simulink model "P1_ADR"  (R2020b)
settings: Solver=VariableStepAuto  StartTime=0.0  StopTime=40  RelTol=1e-3
undefined symbols (not defined in the file): DiscIntNeverNeededParam
libraries: simulink x1
settings Model: Creator=marta  LastModifiedBy=Danie

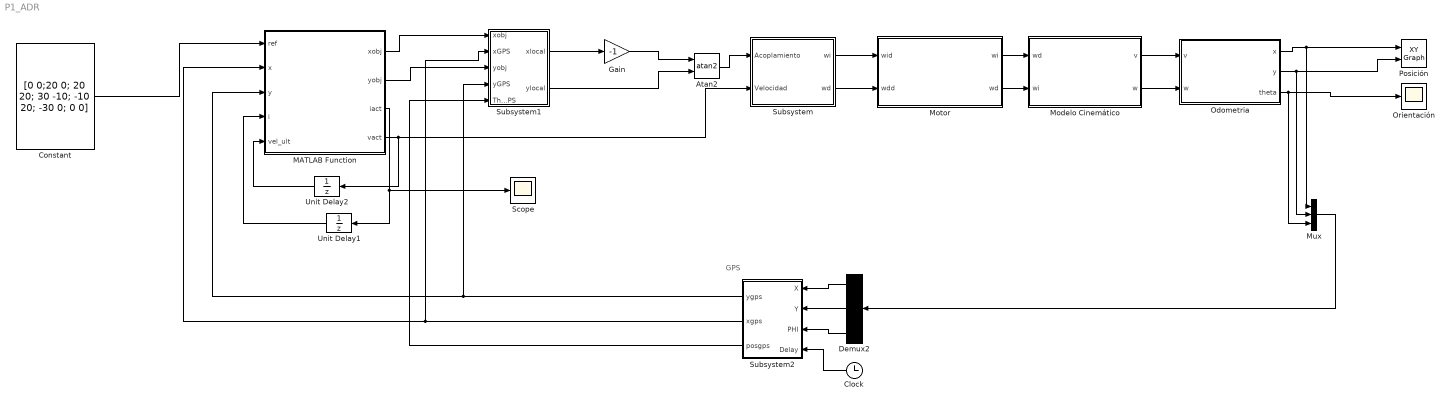
== system P1_ADR ==
  note: GPS
  Atan2 : Trigonometry  Operator=atan2
  Clock : Clock
  Constant : Constant  Value=[0 0;20 0; 20 20; 30 -10; -10 20; -30 0; 0 0]
  Demux2 : Demux  Outputs=3
  Gain : Gain  Gain=-1
  MATLAB Function : MATLAB Function  TreatAsAtomicUnit=on
  Modelo Cinemático : Subsystem
  Motor : Subsystem
  Mux : Mux  Inputs=3
  Odometria : Subsystem
  Orientación : Scope
  Posición : simulink/Sinks/XY Graph  xmin=-5  xmax=5  ymin=-40  ymax=40  st=-1
  Scope : Scope
  Subsystem : Subsystem
  Subsystem1 : Subsystem
  Subsystem2 : Subsystem
  Unit Delay1 : UnitDelay  SampleTime=-1  HasFrameUpgradeWarning=on
  Unit Delay2 : UnitDelay  SampleTime=-1  HasFrameUpgradeWarning=on
  wires:
  Modelo Cinemático/1(v) -> Odometria/1(v)
  Motor/1(wi) -> Modelo Cinemático/1(wd)
  Motor/2(wd) -> Modelo Cinemático/2(wi)
  Modelo Cinemático/2(w) -> Odometria/2(w)
  Odometria/1(x) -> Mux/1, Posición/1
  Odometria/2(y) -> Mux/2, Posición/2
  Odometria/3(theta) -> Mux/3, Orientación/1
  Constant/1 -> MATLAB Function/1(ref)
  MATLAB Function/3(iact) -> Unit Delay1/1, Scope/1
  Unit Delay1/1 -> MATLAB Function/4(i)
  MATLAB Function/1(xobj) -> Subsystem1/1(xobj)
  MATLAB Function/2(yobj) -> Subsystem1/3(yobj)
  Subsystem1/2(ylocal) -> Atan2/2
  Gain/1 -> Atan2/1
  Subsystem1/1(xlocal) -> Gain/1
  Atan2/1 -> Subsystem/1(Acoplamiento)
  Subsystem/2(wd) -> Motor/2(wdd)
  Subsystem/1(wi) -> Motor/1(wid)
  Mux/1 -> Demux2/1
  Demux2/1 -> Subsystem2/1(X)
  Demux2/2 -> Subsystem2/2(Y)
  Demux2/3 -> Subsystem2/3(PHI)
  Clock/1 -> Subsystem2/4(Delay)
  Subsystem2/3(posgps) -> Subsystem1/5(ThetaGPS)
  Subsystem2/2(xgps) -> MATLAB Function/2(x), Subsystem1/2(xGPS)
  Subsystem2/1(ygps) -> MATLAB Function/3(y), Subsystem1/4(yGPS)
  MATLAB Function/4(vact) -> Unit Delay2/1, Subsystem/2(Velocidad)
  Unit Delay2/1 -> MATLAB Function/5(vel_ult)

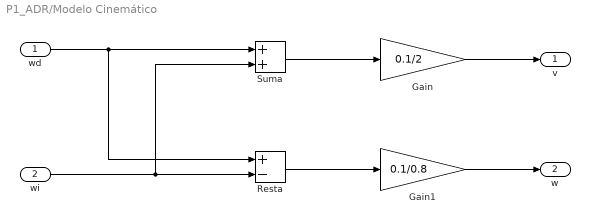
== system P1_ADR/Modelo Cinemático ==
  wd : Inport
  wi : Inport  Port=2
  Gain : Gain  Gain=0.1/2
  Gain1 : Gain  Gain=0.1/0.8
  Resta : Sum  Inputs=+-
  Suma : Sum
  v : Outport
  w : Outport  Port=2
  wires:
  wd/1 -> Resta/1, Suma/1
  Gain/1 -> v/1
  Suma/1 -> Gain/1
  wi/1 -> Resta/2, Suma/2
  Resta/1 -> Gain1/1
  Gain1/1 -> w/1

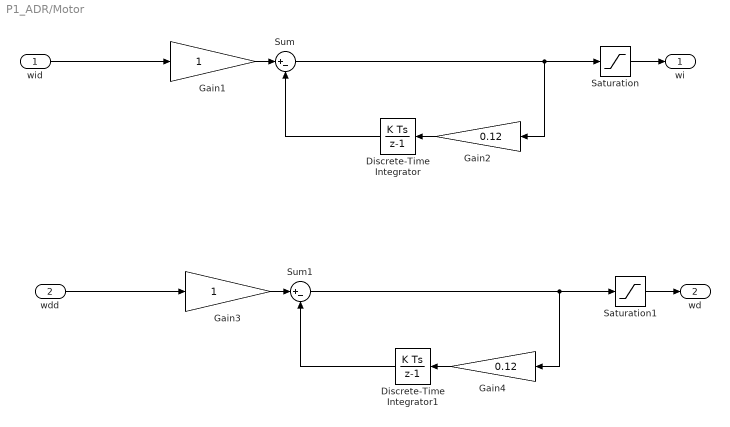
== system P1_ADR/Motor ==
  wid : Inport
  wdd : Inport  Port=2
  Discrete-Time Integrator : DiscreteIntegrator  SampleTime=-1  ICPrevOutput=DiscIntNeverNeededParam  ICPrevScaledInput=DiscIntNeverNeededParam
  Discrete-Time Integrator1 : DiscreteIntegrator  SampleTime=-1  ICPrevOutput=DiscIntNeverNeededParam  ICPrevScaledInput=DiscIntNeverNeededParam
  Gain1 : Gain
  Gain2 : Gain  Gain=0.12
  Gain3 : Gain
  Gain4 : Gain  Gain=0.12
  Saturation : Saturate  UpperLimit=15  LowerLimit=-15
  Saturation1 : Saturate  UpperLimit=15  LowerLimit=-15
  Sum : Sum  Inputs=|+-
  Sum1 : Sum  Inputs=|+-
  wi : Outport
  wd : Outport  Port=2
  wires:
  wid/1 -> Gain1/1
  Gain2/1 -> Discrete-Time Integrator/1
  Saturation/1 -> wi/1
  Gain1/1 -> Sum/1
  Discrete-Time Integrator/1 -> Sum/2
  Sum/1 -> Saturation/1, Gain2/1
  Sum1/1 -> Saturation1/1, Gain4/1
  Discrete-Time Integrator1/1 -> Sum1/2
  Saturation1/1 -> wd/1
  Gain3/1 -> Sum1/1
  Gain4/1 -> Discrete-Time Integrator1/1
  wdd/1 -> Gain3/1

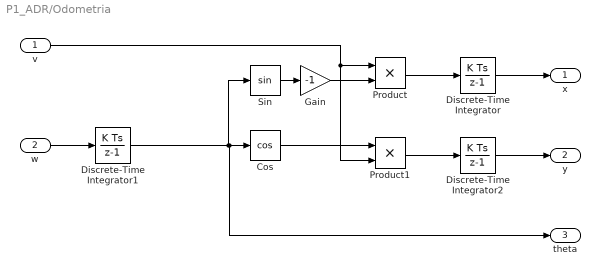
== system P1_ADR/Odometria ==
  v : Inport
  w : Inport  Port=2
  Cos : Trigonometry  Operator=cos
  Discrete-Time Integrator : DiscreteIntegrator  SampleTime=-1  ICPrevOutput=DiscIntNeverNeededParam  ICPrevScaledInput=DiscIntNeverNeededParam
  Discrete-Time Integrator1 : DiscreteIntegrator  SampleTime=-1  ICPrevOutput=DiscIntNeverNeededParam  ICPrevScaledInput=DiscIntNeverNeededParam
  Discrete-Time Integrator2 : DiscreteIntegrator  SampleTime=-1  ICPrevOutput=DiscIntNeverNeededParam  ICPrevScaledInput=DiscIntNeverNeededParam
  Gain : Gain  Gain=-1
  Product : Product
  Product1 : Product
  Sin : Trigonometry
  x : Outport
  y : Outport  Port=2
  theta : Outport  Port=3
  wires:
  Gain/1 -> Product/2
  Product/1 -> Discrete-Time Integrator/1
  Sin/1 -> Gain/1
  v/1 -> Product1/2, Product/1
  Discrete-Time Integrator/1 -> x/1
  Discrete-Time Integrator1/1 -> Sin/1, theta/1, Cos/1
  Cos/1 -> Product1/1
  Product1/1 -> Discrete-Time Integrator2/1
  w/1 -> Discrete-Time Integrator1/1
  Discrete-Time Integrator2/1 -> y/1

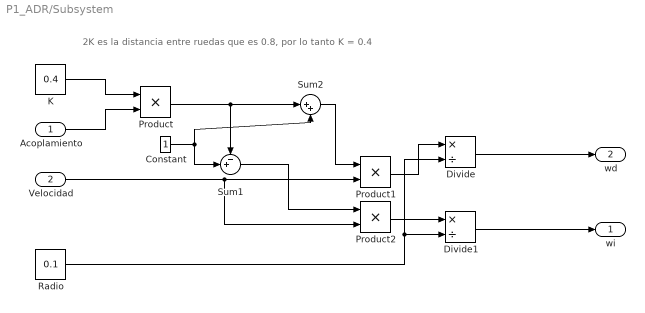
== system P1_ADR/Subsystem ==
  note: 2K es la distancia entre ruedas que es 0.8, por lo tanto K = 0.4
  Acoplamiento : Inport
  Velocidad : Inport  Port=2
  Constant : Constant
  Divide : Product  Inputs=*/
  Divide1 : Product  Inputs=*/
  K : Constant  Value=0.4
  Product : Product
  Product1 : Product
  Product2 : Product
  Radio : Constant  Value=0.1
  Sum1 : Sum  Inputs=-+|
  Sum2 : Sum  Inputs=|++
  wi : Outport
  wd : Outport  Port=2
  wires:
  Divide/1 -> wd/1
  K/1 -> Product/1
  Acoplamiento/1 -> Product/2
  Constant/1 -> Sum2/2, Sum1/2
  Product/1 -> Sum1/1, Sum2/1
  Sum2/1 -> Product1/1
  Velocidad/1 -> Product2/2, Product1/2
  Sum1/1 -> Product2/1
  Product1/1 -> Divide/1
  Radio/1 -> Divide1/2, Divide/2
  Product2/1 -> Divide1/1
  Divide1/1 -> wi/1

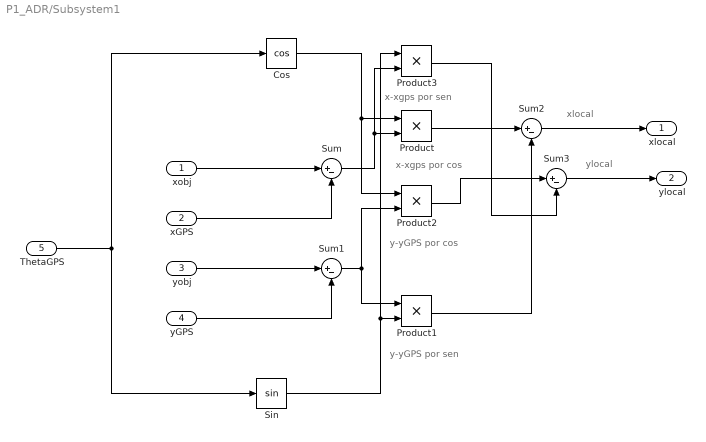
== system P1_ADR/Subsystem1 ==
  note: ylocal
  note: xlocal
  note: y-yGPS por cos
  note: x-xgps por sen
  note: x-xgps por cos
  note: y-yGPS por sen
  xobj : Inport
  xGPS : Inport  Port=2
  yobj : Inport  Port=3
  yGPS : Inport  Port=4
  ThetaGPS : Inport  Port=5
  Cos : Trigonometry  Operator=cos
  Product{,1..3} (4 alike) : Product
  Sin : Trigonometry
  Sum{,1..3} (4 alike) : Sum  Inputs=|+-
  xlocal : Outport
  ylocal : Outport  Port=2
  wires:
  yGPS/1 -> Sum1/2
  yobj/1 -> Sum1/1
  xGPS/1 -> Sum/2
  xobj/1 -> Sum/1
  Sum/1 -> Product3/2, Product/2
  Cos/1 -> Product2/1, Product/1
  ThetaGPS/1 -> Sin/1, Cos/1
  Sin/1 -> Product1/2, Product3/1
  Sum1/1 -> Product1/1, Product2/2
  Product/1 -> Sum2/1
  Product1/1 -> Sum2/2
  Product3/1 -> Sum3/2
  Product2/1 -> Sum3/1
  Sum3/1 -> ylocal/1
  Sum2/1 -> xlocal/1

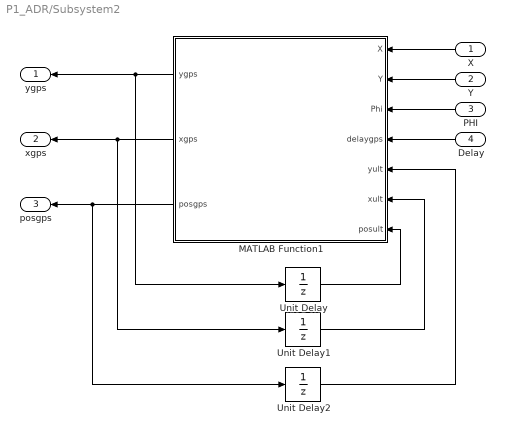
== system P1_ADR/Subsystem2 ==
  X : Inport
  Y : Inport  Port=2
  PHI : Inport  Port=3
  Delay : Inport  Port=4
  MATLAB Function1 : MATLAB Function  TreatAsAtomicUnit=on
  Unit Delay : UnitDelay  SampleTime=-1  HasFrameUpgradeWarning=on
  Unit Delay1 : UnitDelay  SampleTime=-1  HasFrameUpgradeWarning=on
  Unit Delay2 : UnitDelay  SampleTime=-1  HasFrameUpgradeWarning=on
  ygps : Outport
  xgps : Outport  Port=2
  posgps : Outport  Port=3
  wires:
  MATLAB Function1/2(xgps) -> Unit Delay1/1, xgps/1
  MATLAB Function1/3(posgps) -> Unit Delay2/1, posgps/1
  MATLAB Function1/1(ygps) -> Unit Delay/1, ygps/1
  X/1 -> MATLAB Function1/1(X)
  Y/1 -> MATLAB Function1/2(Y)
  PHI/1 -> MATLAB Function1/3(Phi)
  Delay/1 -> MATLAB Function1/4(delaygps)
  Unit Delay/1 -> MATLAB Function1/7(posult)
  Unit Delay1/1 -> MATLAB Function1/6(xult)
  Unit Delay2/1 -> MATLAB Function1/5(yult)

== matlab function P1_ADR/MATLAB Function ==
  data: ref input; x input; xobj output; y input; yobj output; i input; iact output; vact output; vel_ult input
function [xobj, yobj, iact, vact] = sel(ref,x,y,i,vel_ult)
iact=i;
tam=size(ref);
M=tam(1);
xn=ref((iact+1),1)-x;
yn=ref(1,(iact+1))-y;
dist=sqrt(xn^2+yn^2);
vact=vel_ult;

if dist<1
    iact=i+1;
    vact=1.2;
end
if iact+1>M
    iact=M-1;
    vact=0;
end

xobj=ref((iact+1),1);
yobj=ref(1, (iact +1));

end

== matlab function P1_ADR/Subsystem2/MATLAB Function1 ==
  data: X input; ygps output; Y input; Phi input; xgps output; posgps output; delaygps input; yult input; xult input; posult input
function [ygps, xgps, posgps] = GPS(X, Y, Phi, delaygps, yult, xult, posult)

pos=[X; Y; Phi]+sqrtm([0.4 -0.014 0; -0.014 0.5 0; 0 0 0.1])*randn(3,1);
if(mod(delaygps,0.3)==0)
          xgps=real(pos(1));
          ygps=real(pos(2));
          posgps=real(pos(3));
       
else 
          xgps=xult;
          ygps=yult;
          posgps=posult;
          
end
